simulink model "px4demo_read_uorb_example"  (R2017b)
settings: Solver=FixedStepDiscrete  StartTime=0.0  StopTime=inf  FixedStep=0.01  RelTol=1e-3  EnableMultiTasking=on
libraries: pixhawk_slib_uORB_RW x1
Description:
  | PX4 PSP Demo Model - uORB Read
  | 
  | This block is used to read from uORB topics. Open the block and specify a uORB name such as 'sensor_combined'.
  | 
  | Used the buttons on the right to open the .msg file assosciated with the uORB topic to see the variables
  | in the topic structure. Please ensure matching variable structure names, data types and dimension or the generated
  | code will fail to compile
  | 
  | NOTE: This model is to be demosntrated in external mode.
  | An alternative to being able to view these values without external mode is to modify this example to print the signals to the Nuttshell terminal using the print block
settings Model: SimulationMode=external  Creator=darenlee  LastModifiedBy=skuznick
settings DataIOCC: LimitDataPoints=on  SaveFormat=StructureWithTime
settings OptimizationCC: DefaultParameterBehavior=Inlined  LifeSpan=1  MaxStackSize=64
settings DebuggingCC: AllowSymbolicDim=off  SFUnexpectedBacktrackingDiag=warning  SFNoUnconditionalDefaultTransitionDiag=warning  SFExecutionAtInitializationDiag=none
settings HardwareCC: ProdBitPerPointer=32  ProdBitPerSizeT=32  ProdBitPerPtrDiffT=32  ProdLargestAtomicInteger=Long  ProdLargestAtomicFloat=Double  ProdWordSize=32  ProdHWDeviceType=ARM Compatible->ARM Cortex
settings ModelReferenceCC: PropagateSignalLabelsOutOfModel=off
settings SFSimCC: MATLABDynamicMemAlloc=off
settings RTWCC: SystemTargetFile=ert.tlc  HardwareBoard=Pixhawk PX4  TemplateMakefile=ert_default_tmf  GenerateReport=on  Toolchain=Pixhawk Toolchain  IncludeHyperlinkInReport=on  LaunchReport=on  GenerateTraceInfo=on  GenerateTraceReport=on  GenerateTraceReportSl=on  GenerateTraceReportSf=on  GenerateTraceReportEml=on
settings CodeAppCC: IgnoreCustomStorageClasses=off  StateflowObjectComments=on
settings ERTTargetCC: MultiwordLength=2048  ExtMode=on  ExtModeTransport=1  ExtModeMexFile=ext_serial_win32_comm  ExtModeMexArgs=1 4 115200  ERTCustomFileTemplate=px4_codertarget_file_process.tlc  ConvertIfToSwitch=off  SuppressUnreachableDefaultCases=off
settings ConfigComp: CovMetricSettings=dw  CovHtmlReporting=on  CovSaveCumulativeToWorkspaceVar=on  CovSaveSingleToWorkspaceVar=on  CovExternalEMLEnable=off

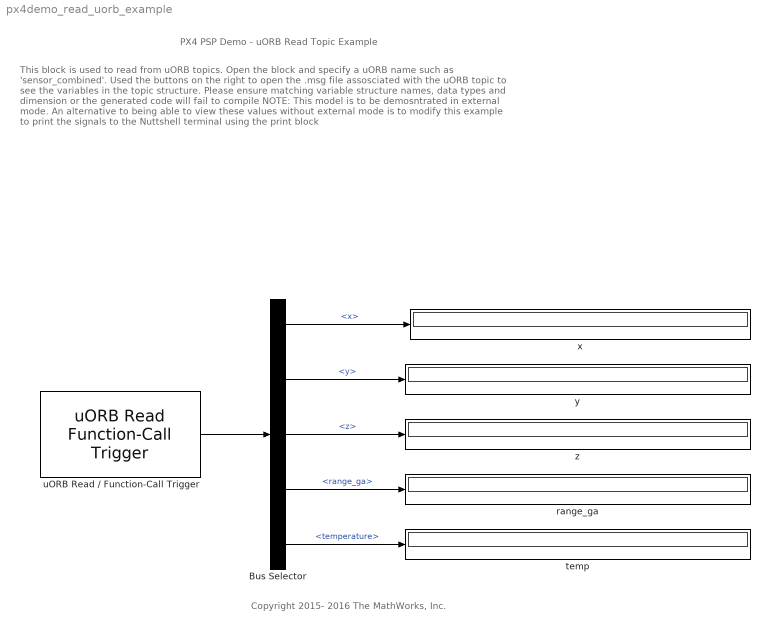
== system px4demo_read_uorb_example ==
  note: PX4 PSP Demo - uORB Read Topic Example
  note: This block is used to read from uORB topics. Open the block and specify a uORB name such as 'sensor_combined'.
      |
      | Used the buttons on the right to open the .msg file assosciated with the uORB topic to see the variables
      | in the topic structure. Please ensure matching variable structure names, data types and dimension or the generated
      | code will fail to compile
      |
      | NOTE: This model is to be demosntrated in external mode.
      | An alternative to being able to view these values without external mode is to modify this example to print the signals to the Nuttshell terminal using the print block
  note: Copyright 2015- 2016 The MathWorks, Inc.
  Bus Selector : BusSelector  OutputSignals=x,y,z,range_ga,temperature
  range_ga : Display
  temp : Display
  uORB Read / Function-Call Trigger : pixhawk_slib_uORB_RW/uORB Read Function-Call Trigger  uORB_Topic_str='sensor_mag'  BusObjVar=Bus: sensor_mag_SL  uORB_Interval=1  AsyncOutput=off  Fcn_call_select=Generate Function Call Signal  TaskName='Task1'  Poll_timeout=100  Ts=-1
      settings: SourceProductName=Pixhawk Target Blocks
  x : Display
  y : Display
  z : Display
  wires:
  Bus Selector/1 -> x/1  "<x>"
  Bus Selector/2 -> y/1  "<y>"
  Bus Selector/3 -> z/1  "<z>"
  Bus Selector/4 -> range_ga/1  "<range_ga>"
  Bus Selector/5 -> temp/1  "<temperature>"
  uORB Read / Function-Call Trigger/1 -> Bus Selector/1
